simulink model "Water_Transport"  (R2021b)
settings: Solver=VariableStepAuto  StartTime=0.0  StopTime=10.0  RelTol=1e-3
settings Model: Creator=CYY-WS-021  LastModifiedBy=CYY-WS-021

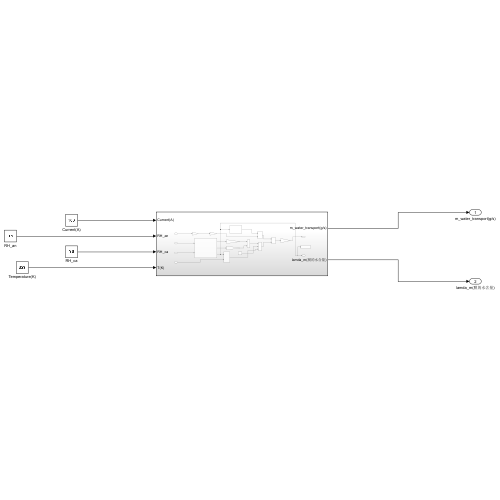
[thumbnail: Simulink's stored preview of the top-level diagram]
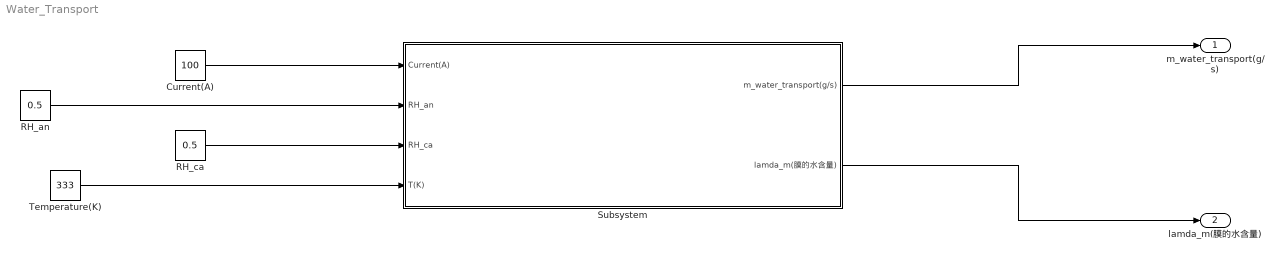
== system Water_Transport ==
  Current(A) : Constant  Value=100
  RH_an : Constant  Value=0.5
  RH_ca : Constant  Value=0.5
  Subsystem : Subsystem
  Temperature(K) : Constant  Value=333
  m_water_transport(g/s) : Outport
  lamda_m(膜的水含量) : Outport  Port=2
  wires:
  Current(A)/1 -> Subsystem/1(Current(A))
  RH_an/1 -> Subsystem/2(RH_an)
  RH_ca/1 -> Subsystem/3(RH_ca)
  Temperature(K)/1 -> Subsystem/4(T(K))
  Subsystem/1(m_water_transport(g/s)) -> m_water_transport(g/s)/1
  Subsystem/2(lamda_m(膜的水含量)) -> lamda_m(膜的水含量)/1

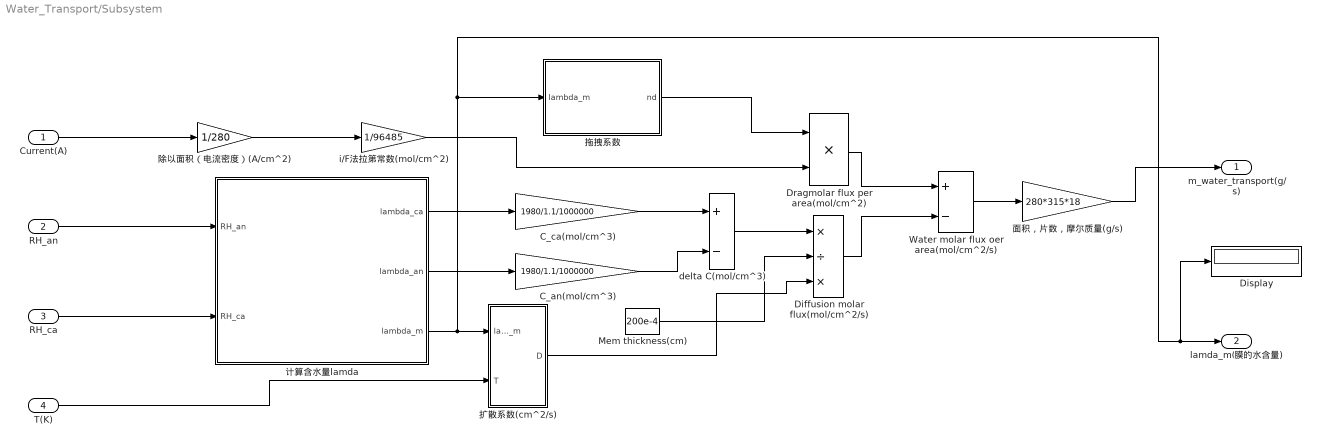
== system Water_Transport/Subsystem ==
  Current(A) : Inport
  RH_an : Inport  Port=2
  RH_ca : Inport  Port=3
  T(K) : Inport  Port=4
  "\tC_an(mol/cm^3)" : Gain  Gain=1980/1.1/1000000
  "\tC_ca(mol/cm^3)" : Gain  Gain=1980/1.1/1000000
  Diffusion molar flux(mol/cm^2/s) : Product  Inputs=*/*
  Display : Display
  Dragmolar flux per area(mol/cm^2) : Product
  Mem thickness(cm) : Constant  Value=200e-4
  Water molar flux oer area(mol/cm^2/s) : Sum  Inputs=+-
  delta C(mol/cm^3) : Sum  Inputs=+-
  i/F法拉第常数(mol/cm^2) : Gain  Gain=1/96485
  扩散系数(cm^2/s) : MATLAB Function  TreatAsAtomicUnit=on
  拖拽系数 : MATLAB Function  TreatAsAtomicUnit=on
  计算含水量lamda : MATLAB Function  TreatAsAtomicUnit=on
  除以面积（电流密度）(A/cm^2) : Gain  Gain=1/280
  面积，片数，摩尔质量(g/s) : Gain  Gain=280*315*18
  m_water_transport(g/s) : Outport
  lamda_m(膜的水含量) : Outport  Port=2
  wires:
  除以面积（电流密度）(A/cm^2)/1 -> i/F法拉第常数(mol/cm^2)/1
  计算含水量lamda/1(lambda_ca) -> "\tC_ca(mol/cm^3)"/1
  计算含水量lamda/3(lambda_m) -> lamda_m(膜的水含量)/1, Display/1, 拖拽系数/1(lambda_m), 扩散系数(cm^2/s)/1(lamda_m)
  Diffusion molar flux(mol/cm^2/s)/1 -> Water molar flux oer area(mol/cm^2/s)/2
  Mem thickness(cm)/1 -> Diffusion molar flux(mol/cm^2/s)/2
  扩散系数(cm^2/s)/1(D) -> Diffusion molar flux(mol/cm^2/s)/3
  "\tC_an(mol/cm^3)"/1 -> delta C(mol/cm^3)/2
  Dragmolar flux per area(mol/cm^2)/1 -> Water molar flux oer area(mol/cm^2/s)/1
  Water molar flux oer area(mol/cm^2/s)/1 -> 面积，片数，摩尔质量(g/s)/1
  拖拽系数/1(nd) -> Dragmolar flux per area(mol/cm^2)/1
  i/F法拉第常数(mol/cm^2)/1 -> Dragmolar flux per area(mol/cm^2)/2
  delta C(mol/cm^3)/1 -> Diffusion molar flux(mol/cm^2/s)/1
  计算含水量lamda/2(lambda_an) -> "\tC_an(mol/cm^3)"/1
  "\tC_ca(mol/cm^3)"/1 -> delta C(mol/cm^3)/1
  面积，片数，摩尔质量(g/s)/1 -> m_water_transport(g/s)/1
  T(K)/1 -> 扩散系数(cm^2/s)/2(T)
  Current(A)/1 -> 除以面积（电流密度）(A/cm^2)/1
  RH_an/1 -> 计算含水量lamda/1(RH_an)
  RH_ca/1 -> 计算含水量lamda/2(RH_ca)

== matlab function Water_Transport/Subsystem/扩散系数(cm^2//s) ==
  data: lamda_m input; D output; T input
function D = fcn(lamda_m,T)
if lamda_m<2
    D=1e-6*exp(2416*(1/303-1/T));

elseif lamda_m>=2 && lamda_m<3
    D=1e-6*(1+(2*lamda_m-2))*exp(2416*(1/303-1/T));
elseif lamda_m>=3 && lamda_m<=4.5
    D=1e-6*(3-(1.67*lamda_m-3))*exp(2416*(1/303-1/T));
else 
    D=1.25e-6*exp(2416*(1/303-1/T));
end

== matlab function Water_Transport/Subsystem/计算含水量lamda ==
  data: RH_an input; lambda_ca output; RH_ca input; lambda_an output; lambda_m output
function [lambda_ca,lambda_an,lambda_m]= fcn(RH_an,RH_ca)
if RH_an>=1
    lambda_an=14+1.4*(RH_an-1);
else lambda_an=0.043+17.81*RH_an-39.85*RH_an^2+36*RH_an^3;
end
if RH_ca>=1
    lambda_ca=14+1.4*(RH_ca-1);
else lambda_ca=0.043+17.81*RH_ca-39.85*RH_ca^2+36*RH_ca^3;
end
RH_m = 0.5*(RH_ca+RH_an);
if RH_m>=1
    lambda_m=14+1.4*(RH_m-1);
else lambda_m=0.043+17.81*RH_m-39.85*RH_m^2+36*RH_m^3;
end

== matlab function Water_Transport/Subsystem/拖拽系数 ==
  data: lambda_m input; nd output
function nd= fcn(lambda_m)

nd=0.0029*lambda_m^2+0.05/lambda_m-3.4e-19;
